simulink model "a3_system_2"  (Simulink 7.3)
settings: Solver=ode45  StartTime=0.0  StopTime=10.0  RelTol=1e-3
libraries: simulink_extras x2
Description:
  | Takes as input [m, l2, g]
settings Model: Creator=Tarik  LastModifiedBy=Tarik

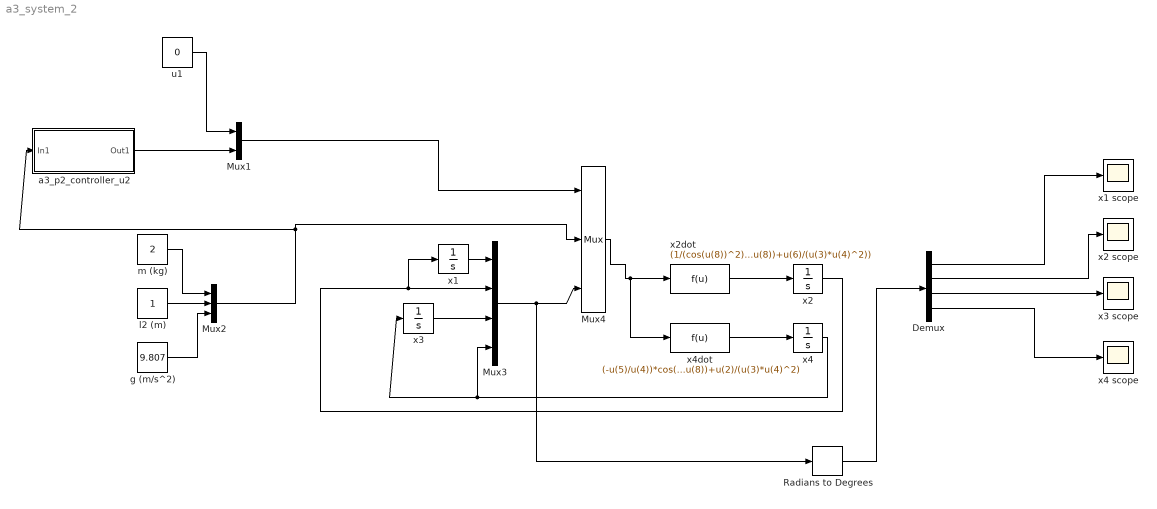
== system a3_system_2 ==
  Demux : Demux
  Mux1 : Mux  Inputs=2
  Mux2 : Mux  Inputs=3
  Mux3 : Mux
  Mux4 : Mux  Description=|  Inputs=3
      | u(1:2) are u1 and u2   
      | u(3:5) are m, l2, and g
      | u(6:9) are x1 x2 x3 x4
  Radians to Degrees : simulink_extras/Transformations/Radians to Degrees  SystemSampleTime=-1
  a3_p2_controller_u2 : Subsystem  Description=Input is properties (m l g)
  g (m/s^2) : Constant  Value=9.807  OutDataType=fixdt(1, 16)  OutScaling=2^0
  l2 (m) : Constant  OutDataType=fixdt(1, 16)  OutScaling=2^0
  m (kg) : Constant  Value=2  OutDataType=fixdt(1, 16)  OutScaling=2^0
  u1 : Constant  Value=0  OutDataType=fixdt(1, 16)  OutScaling=2^0
  x1 : Integrator
  x1 scope : Scope
  x2 : Integrator
  x2 scope : Scope
  x2dot : Fcn  Expr=(1/(cos(u(8))^2))*(u(7)*u(9)*sin(2*u(8))+u(6)/(u(3)*u(4)^2))
  x3 : Integrator  InitialCondition=pi/4
  x3 scope : Scope
      settings: SaveName=ScopeData2
  x4 : Integrator
  x4 scope : Scope
      settings: SaveName=ScopeData3
  x4dot : Fcn  Expr=(-u(5)/u(4))*cos(u(8))-(u(7)/2)*sin(2*u(8))+u(2)/(u(3)*u(4)^2)
  wires:
  Demux/1 -> x1 scope/1
  Demux/2 -> x2 scope/1
  Demux/3 -> x3 scope/1
  Demux/4 -> x4 scope/1
  m (kg)/1 -> Mux2/1
  l2 (m)/1 -> Mux2/2
  g (m/s^2)/1 -> Mux2/3
  x2dot/1 -> x2/1
  x4dot/1 -> x4/1
  x1/1 -> Mux3/1
  Mux3/1 -> Mux4/3, Radians to Degrees/1
  Mux2/1 -> Mux4/2, a3_p2_controller_u2/1(In1)
  Mux1/1 -> Mux4/1
  Mux4/1 -> x2dot/1, x4dot/1
  Radians to Degrees/1 -> Demux/1
  u1/1 -> Mux1/1
  a3_p2_controller_u2/1(Out1) -> Mux1/2
  x3/1 -> Mux3/3
  x4/1 -> Mux3/4, x3/1
  x2/1 -> Mux3/2, x1/1

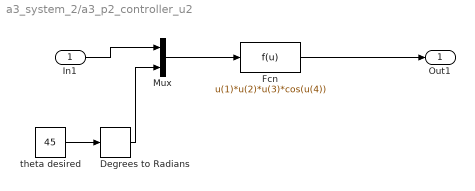
== system a3_system_2/a3_p2_controller_u2 ==
  In1 : Inport  PortDimensions=3  OutDataType=fixdt(1, 16)  OutScaling=2^0
  Degrees to Radians : simulink_extras/Transformations/Degrees to Radians  SystemSampleTime=-1
  Fcn : Fcn  Expr=u(1)*u(2)*u(3)*cos(u(4))
  Mux : Mux  Inputs=2
  theta desired : Constant  Value=45  OutDataType=fixdt(1, 16)  OutScaling=2^0
  Out1 : Outport  OutDataType=fixdt(1, 16)  OutScaling=2^0
  wires:
  Fcn/1 -> Out1/1
  Mux/1 -> Fcn/1
  In1/1 -> Mux/1
  theta desired/1 -> Degrees to Radians/1
  Degrees to Radians/1 -> Mux/2
